simulink model "Subsystem_repository0x5B10x5D"  (R2023b)
settings: Solver=VariableStepAuto  StartTime=0.0  StopTime=10.0  RelTol=1e-3
values from neighbouring files (symbols this model uses):
  A0 = [1 0 0; 0 0 1; 0 -1 0]*[0 0 1; 0 1 0; -1 0 0]    [planetary_phase_script.m]    (also in script_aocs.m = [0 0 1; 0 1 0; -1 0 0]; script_jupiter.m; simulation_inner1.m = A_b_n(:,:,end); srp_interplanetary.m = A_b_n(:,:,end))
  mu = astroConstants(4)    [calcolo_distanze.m]    (also in loadData.m; loadData_ore.m; planetary_phase_script.m = astroConstants(15); script_aocs.m)
  toll = deg2rad(15)    [planetary_phase_script.m]    (also in script_aocs.m; script_jupiter.m; simulation_inner1.m; srp_interplanetary.m)
undefined symbols (not defined in the file or in its folder): N, q0
libraries: simulink x3, matrix_library x3, vrlib x1
(part 1 of 2)
settings Model: Creator=ricky  LastModifiedBy=paolo

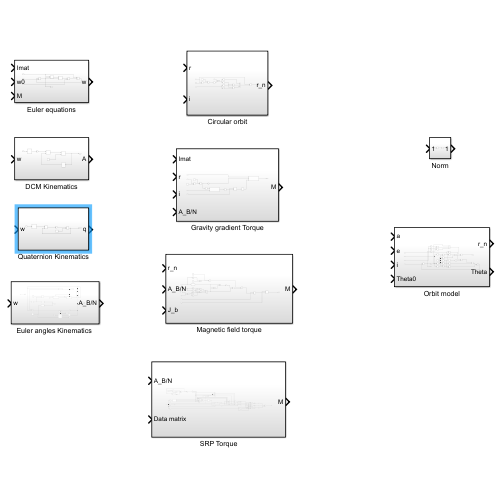
[thumbnail: Simulink's stored preview of the top-level diagram]
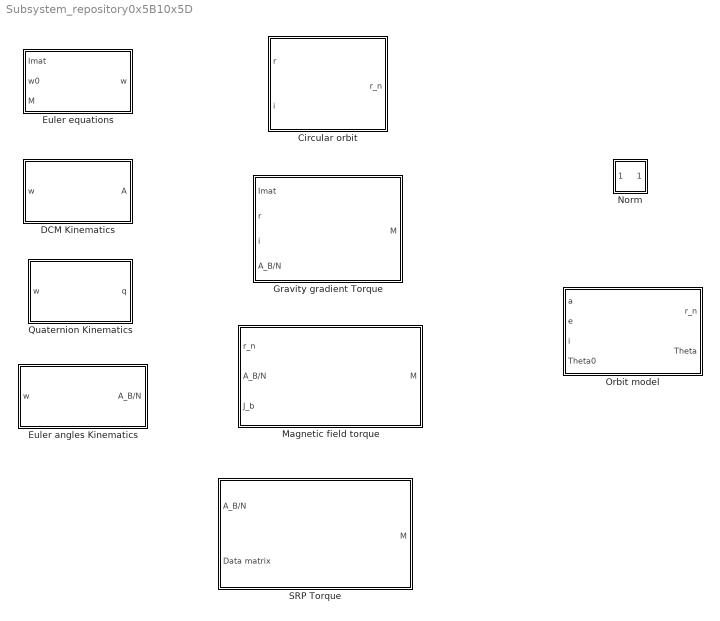
== system Subsystem_repository0x5B10x5D ==
  Circular orbit : Subsystem
  DCM Kinematics : Subsystem
  "Euler angles Kinematics " : Subsystem
  Euler equations : Subsystem
  Gravity gradient Torque : Subsystem
  Magnetic field torque : Subsystem
  Norm : Subsystem
  Orbit model : Subsystem
  Quaternion Kinematics : Subsystem
  SRP Torque : Subsystem

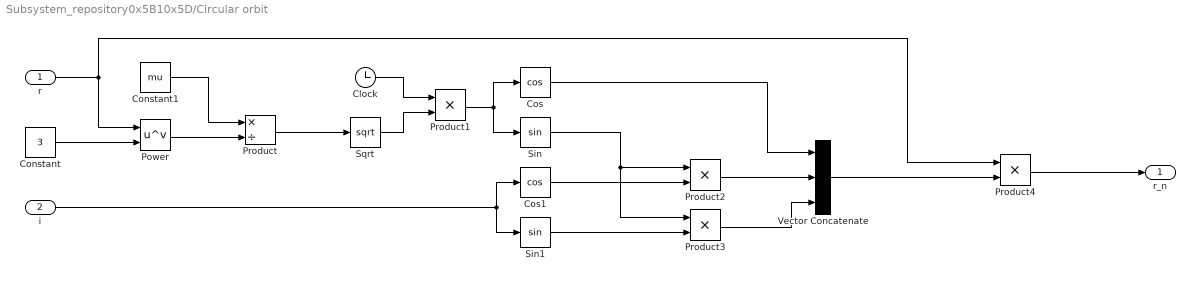
== system Subsystem_repository0x5B10x5D/Circular orbit ==
  r : Inport
  i : Inport  Port=2
  Clock : Clock
  Constant : Constant  Value=3
  Constant1 : Constant  Value=mu
  Cos : Trigonometry  Operator=cos
  Cos1 : Trigonometry  Operator=cos
  Power : Math  Operator=pow
  Product : Product  Inputs=*/
  Product{1..4} (4 alike) : Product
  Sin : Trigonometry
  Sin1 : Trigonometry
  Sqrt : Sqrt
  Vector Concatenate : Concatenate  NumInputs=3
  r_n : Outport
  wires:
  Product/1 -> Sqrt/1
  Constant/1 -> Power/2
  Constant1/1 -> Product/1
  Power/1 -> Product/2
  r/1 -> Product4/1, Power/1
  Clock/1 -> Product1/1
  Sqrt/1 -> Product1/2
  Product1/1 -> Cos/1, Sin/1
  i/1 -> Sin1/1, Cos1/1
  Product2/1 -> Vector Concatenate/2
  Product3/1 -> Vector Concatenate/3
  Cos/1 -> Vector Concatenate/1
  Sin/1 -> Product3/1, Product2/1
  Cos1/1 -> Product2/2
  Sin1/1 -> Product3/2
  Vector Concatenate/1 -> Product4/2
  Product4/1 -> r_n/1

== system Subsystem_repository0x5B10x5D/DCM Kinematics ==
  w : Inport
  Constant : Constant  Value=A0
  Gain : Gain  Gain=-1
  Integrator : Integrator  InitialConditionSource=external
  Matrix Creation : Subsystem
  Matrix orthonormalization : Subsystem
  MatrixMultiply : Product  Multiplication=Matrix(*)
  A : Outport
  wires:
  Matrix orthonormalization/1(Out1) -> MatrixMultiply/2
  Integrator/1 -> A/1, Matrix orthonormalization/1(A)  "A"
  Constant/1 -> Integrator/2
  MatrixMultiply/1 -> Integrator/1  "A_d"
  Matrix Creation/1(Out1) -> Gain/1
  Gain/1 -> MatrixMultiply/1
  w/1 -> Matrix Creation/1(Input)

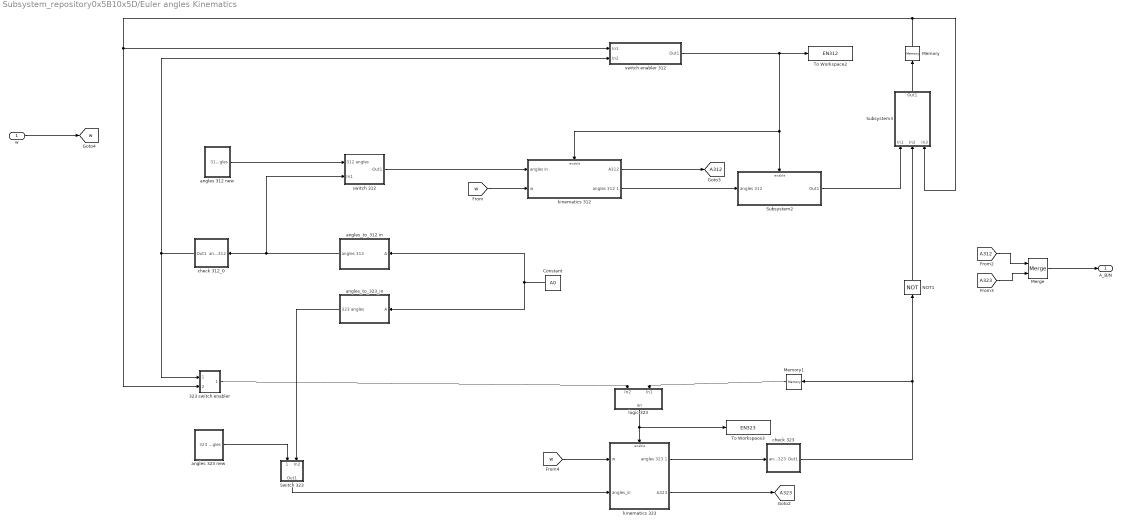
== system Subsystem_repository0x5B10x5D/Euler angles Kinematics  ==
  w : Inport
  323 switch enabler : Subsystem
  Constant : Constant  Value=A0
  Memory : Memory  InheritSampleTime=on
  Memory1 : Memory
  Merge : Merge
  NOT1 : Logic  Operator=NOT  IconShape=distinctive  AllPortsSameDT=off  OutDataTypeStr=boolean
  Subsystem2 : Subsystem
  Subsystem3 : Subsystem
  Switch 323 : Subsystem
  To Workspace2 : ToWorkspace  VariableName=EN312  SampleTime=-1
  To Workspace3 : ToWorkspace  VariableName=EN323  SampleTime=-1
  angles 312 new : Subsystem
  angles 323 new : Subsystem
  angles_to_312 in : Subsystem
  angles_to_323_in : Subsystem
  check 312_0 : Subsystem
      settings: PortSchema="{\"entries\":[{\"content\":{\"sides\":[{\"content\":{},\"type\":\"ConnectorPlacement.EquallySpacedRectSide\",\"uuid\":\"ce510fac-c30a-4239-a3ca-34d3b3a25917\"},{\"content\":{\"side\":\"RIGHT\"},\"type\":\"ConnectorPlacement.EquallySpacedRectSide\",\"uuid\":\"eef8e0af-d591-4c9d-a699-4633d685d136\"},{\"content\":{\"connectorIds\":[\"Out1\"],\"side\":\"TOP\"},\"type\":\"ConnectorPlacement.EquallySpacedRectSide\",\"uuid\":\"fcaa08d0-a3a1-4dce-b64a-8b5dfd06733d\"},{\"content\":{\"connectorIds\":[\"In1\"],\"side\":\"BOTTOM\"},\"type\":\"ConnectorPlacement.EquallySpacedRectSide\",\"uuid\":\"e9ea2ab9-2ba0-4219-9d61-f42bbc501f13\"}]},\"type\":\"ConnectorPlacement.EquallySpacedConnector\",\"uuid\":\"4537d4ba-38a8-4a93-90f3-8d5d5085984b\"}],\"packageUris\":[\"http://schema.mathworks.com/mf0/Connector/R2020b\"],\"version\":\"1.0\"}"
  check 323 : Subsystem
      settings: PortSchema="{\"entries\":[{\"content\":{\"sides\":[{\"content\":{},\"type\":\"ConnectorPlacement.EquallySpacedRectSide\",\"uuid\":\"ce510fac-c30a-4239-a3ca-34d3b3a25917\"},{\"content\":{\"side\":\"RIGHT\"},\"type\":\"ConnectorPlacement.EquallySpacedRectSide\",\"uuid\":\"eef8e0af-d591-4c9d-a699-4633d685d136\"},{\"content\":{\"connectorIds\":[\"Out1\"],\"side\":\"TOP\"},\"type\":\"ConnectorPlacement.EquallySpacedRectSide\",\"uuid\":\"fcaa08d0-a3a1-4dce-b64a-8b5dfd06733d\"},{\"content\":{\"connectorIds\":[\"In1\"],\"side\":\"BOTTOM\"},\"type\":\"ConnectorPlacement.EquallySpacedRectSide\",\"uuid\":\"e9ea2ab9-2ba0-4219-9d61-f42bbc501f13\"}]},\"type\":\"ConnectorPlacement.EquallySpacedConnector\",\"uuid\":\"4537d4ba-38a8-4a93-90f3-8d5d5085984b\"}],\"packageUris\":[\"http://schema.mathworks.com/mf0/Connector/R2020b\"],\"version\":\"1.0\"}"
  kinematics 312 : Subsystem
  kinematics 323 : Subsystem
  logic 323 : Subsystem
  switch 312 : Subsystem
  switch enabler 312 : Subsystem
  A_B/N : Outport
  tag scope: A312=global, A323=global, w=global
  wires:
  kinematics 323/2(A323) -> [A323]
  Constant/1 -> angles_to_323_in/1(A), angles_to_312 in/1(A)
  323 switch enabler/1(Out1) -> logic 323/1(In2)
  logic 323/1(en) -> To Workspace3/1, kinematics 323/Enable
  switch enabler 312/1(Out1) -> To Workspace2/1, Subsystem2/Enable, kinematics 312/Enable
  kinematics 312/2(angles 312 1) -> Subsystem2/1(angles 312)
  check 312_0/1(Out1) -> switch enabler 312/2(In2), 323 switch enabler/1(In2)
  [w] -> kinematics 323/1(w)
  angles_to_312 in/1(angles 312) -> switch 312/2(In1), check 312_0/1(angles 312)
  Memory1/1 -> logic 323/2(In1)
  Subsystem3/1(Out1) -> Memory/1
  w/1 -> [w]
  NOT1/1 -> Subsystem3/2(In2)
  Memory/1 -> Subsystem3/3(In3), 323 switch enabler/2(In1), switch enabler 312/1(In1)
  kinematics 323/1(angles 323 1) -> check 323/1(angles 323)
  kinematics 312/1(A312) -> [A312]
  switch 312/1(Out1) -> kinematics 312/1(angles in)
  Merge/1 -> A_B/N/1
  Switch 323/1(Out1) -> kinematics 323/2(angles_in)
  check 323/1(Out1) -> NOT1/1, Memory1/1
  Subsystem2/1(Out1) -> Subsystem3/1(In1)
  angles 323 new/1(323 angles) -> Switch 323/1(323 angles)
  angles 312 new/1(312 angles) -> switch 312/1(312 angles)
  [w] -> kinematics 312/2(w)
  angles_to_323_in/1(323 angles) -> Switch 323/2(In2)
  [A323] -> Merge/2
  [A312] -> Merge/1

== system Subsystem_repository0x5B10x5D/Euler equations ==
  Imat : Inport
  w0 : Inport  Port=2
  M : Inport  Port=3
  Cross Product : matrix_library/Cross Product
  Integrator1 : Integrator  InitialConditionSource=external
  Product : Product  Multiplication=Matrix(*)
  Product1 : Product  Inputs=/*  Multiplication=Matrix(*)
  Subtract : Sum
  w : Outport
  wires:
  Imat/1 -> Product1/1, Product/1
  Integrator1/1 -> w/1, Product/2, Cross Product/2  "w"
  Product/1 -> Cross Product/1
  w0/1 -> Integrator1/2
  Cross Product/1 -> Subtract/1
  M/1 -> Subtract/2
  Subtract/1 -> Product1/2
  Product1/1 -> Integrator1/1

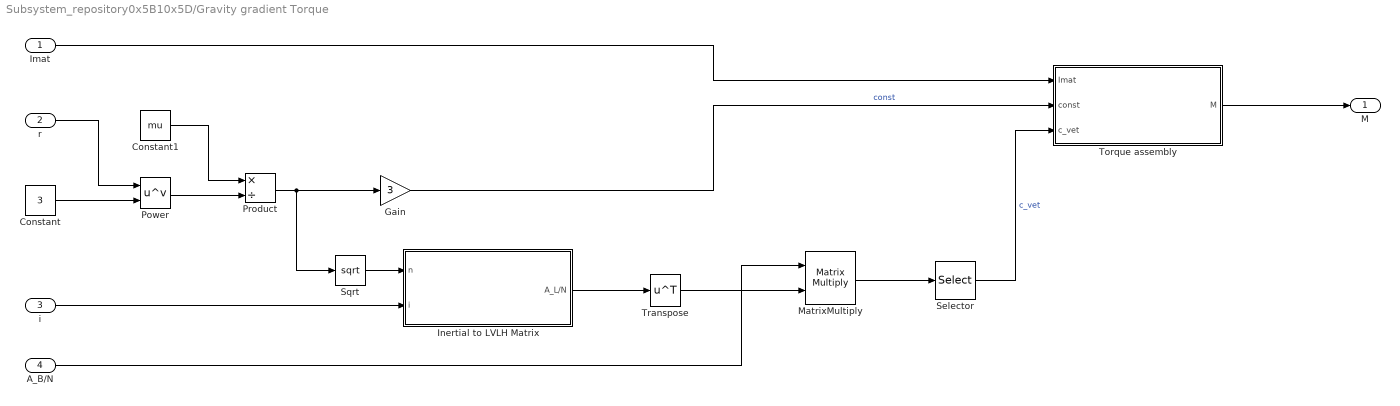
== system Subsystem_repository0x5B10x5D/Gravity gradient Torque ==
  Imat : Inport
  r : Inport  Port=2
  i : Inport  Port=3
  A_B/N : Inport  Port=4
  Constant : Constant  Value=3
  Constant1 : Constant  Value=mu
  Gain : Gain  Gain=3
  Inertial to LVLH Matrix : Subsystem
  MatrixMultiply : Product  Multiplication=Matrix(*)
  Power : Math  Operator=pow
  Product : Product  Inputs=*/
  Selector : Selector  NumberOfDimensions=2  InputPortWidth=3  IndexOptions=Index vector (dialog),Index vector (dialog)  Indices=[1 2 3],1  OutputSizes=1,1
  Sqrt : Sqrt
  Torque assembly : Subsystem
  Transpose : Math  Operator=transpose
  M : Outport
  wires:
  Inertial to LVLH Matrix/1(A_L/N) -> Transpose/1
  Transpose/1 -> MatrixMultiply/2
  MatrixMultiply/1 -> Selector/1
  i/1 -> Inertial to LVLH Matrix/2(i)
  A_B/N/1 -> MatrixMultiply/1
  Power/1 -> Product/2
  r/1 -> Power/1
  Constant/1 -> Power/2
  Product/1 -> Sqrt/1, Gain/1
  Constant1/1 -> Product/1
  Sqrt/1 -> Inertial to LVLH Matrix/1(n)
  Selector/1 -> Torque assembly/3(c_vet)  "c_vet"
  Gain/1 -> Torque assembly/2(const)  "const"
  Imat/1 -> Torque assembly/1(Imat)
  Torque assembly/1(M) -> M/1

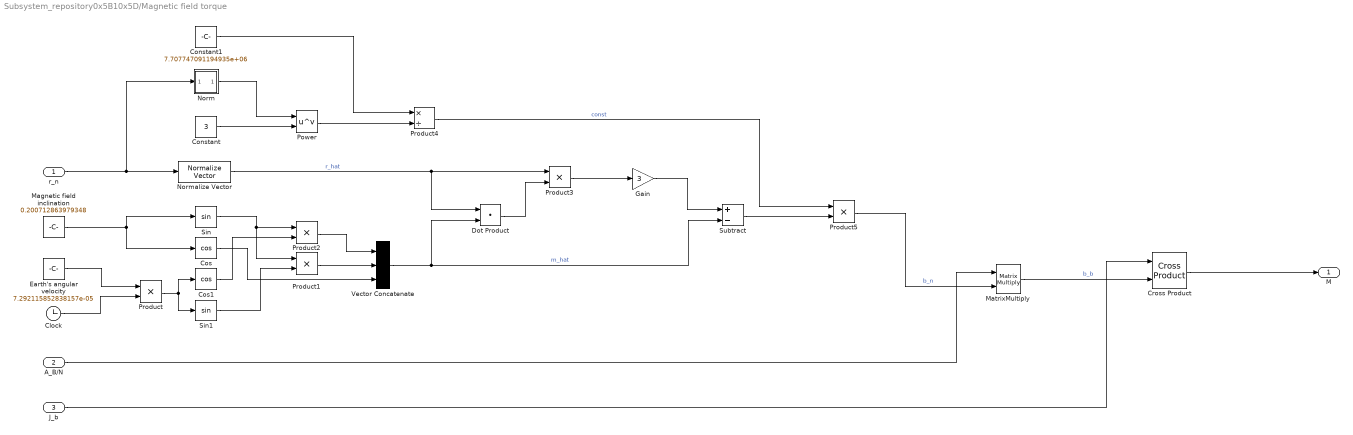
== system Subsystem_repository0x5B10x5D/Magnetic field torque ==
  r_n : Inport
  A_B/N : Inport  Port=2
  J_b : Inport  Port=3
  Clock : Clock
  Constant : Constant  Value=3
  Constant1 : Constant  Value=7.707747091194935e+06
  Cos : Trigonometry  Operator=cos
  Cos1 : Trigonometry  Operator=cos
  Cross Product : matrix_library/Cross Product
  Dot Product : DotProduct  OutDataTypeStr=Inherit: Inherit via internal rule
  Earth's angular velocity : Constant  Value=7.292115852838157e-05
  Gain : Gain  Gain=3
  Magnetic field inclination : Constant  Value=0.200712863979348
  MatrixMultiply : Product  Multiplication=Matrix(*)
  Norm : Subsystem
  Normalize Vector : vrlib/Utilities/Normalize Vector  maxzero=0
  Power : Math  Operator=pow
  Product{,1..3,5} (5 alike) : Product
  Product4 : Product  Inputs=*/
  Sin : Trigonometry
  Sin1 : Trigonometry
  Subtract : Sum  Inputs=+-
  Vector Concatenate : Concatenate  NumInputs=3
  M : Outport
  wires:
  r_n/1 -> Norm/1(1), Normalize Vector/1
  Normalize Vector/1 -> Product3/1, Dot Product/1  "r_hat"
  Earth's angular velocity/1 -> Product/1
  Clock/1 -> Product/2
  Product/1 -> Sin1/1, Cos1/1
  Magnetic field inclination/1 -> Cos/1, Sin/1
  Cos/1 -> Vector Concatenate/3
  Product1/1 -> Vector Concatenate/2
  Product2/1 -> Vector Concatenate/1
  Sin/1 -> Product1/1, Product2/1
  Cos1/1 -> Product2/2
  Sin1/1 -> Product1/2
  Vector Concatenate/1 -> Subtract/2, Dot Product/2  "m_hat"
  Dot Product/1 -> Product3/2
  Product3/1 -> Gain/1
  Gain/1 -> Subtract/1
  A_B/N/1 -> MatrixMultiply/1
  MatrixMultiply/1 -> Cross Product/2  "b_b"
  J_b/1 -> Cross Product/1
  Constant1/1 -> Product4/1
  Subtract/1 -> Product5/2
  Product4/1 -> Product5/1  "const"
  Product5/1 -> MatrixMultiply/2  "b_n"
  Cross Product/1 -> M/1
  Constant/1 -> Power/2
  Power/1 -> Product4/2
  Norm/1(Output) -> Power/1

== system Subsystem_repository0x5B10x5D/Norm ==
  1 : Inport
  Dot Product : DotProduct  OutDataTypeStr=Inherit: Inherit via internal rule
  Sqrt : Sqrt
  Output : Outport
  wires:
  1/1 -> Dot Product/1, Dot Product/2
  Dot Product/1 -> Sqrt/1
  Sqrt/1 -> Output/1

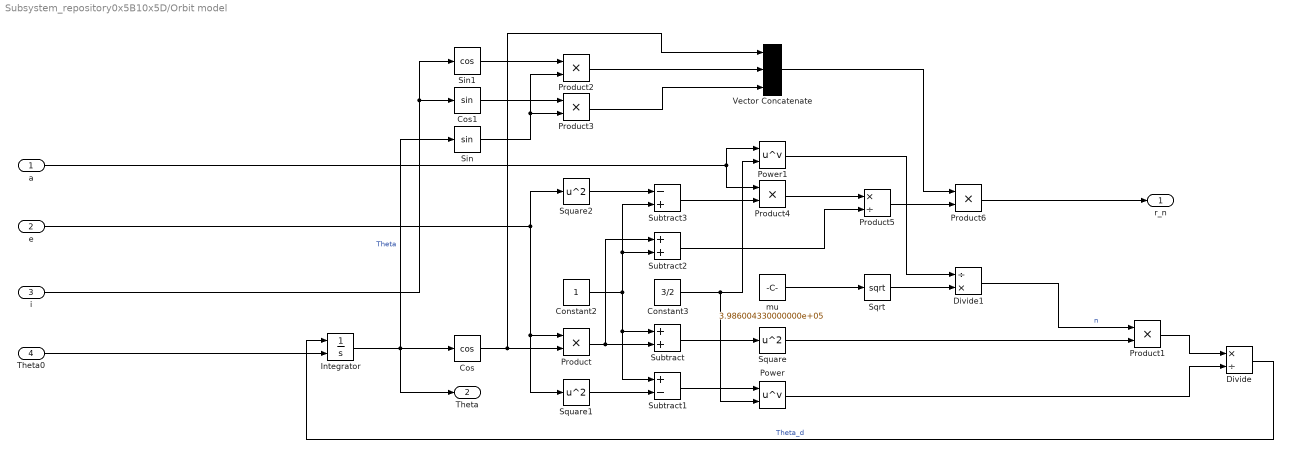
== system Subsystem_repository0x5B10x5D/Orbit model ==
  a : Inport
  e : Inport  Port=2
  i : Inport  Port=3
  Theta0 : Inport  Port=4
  Constant2 : Constant
  Constant3 : Constant  Value=3/2
  Cos : Trigonometry  Operator=cos
  Cos1 : Trigonometry
  Divide : Product  Inputs=*/
  Divide1 : Product  Inputs=/*
  Integrator : Integrator  InitialConditionSource=external
  Power : Math  Operator=pow
  Power1 : Math  Operator=pow
  Product{,1..4,6} (6 alike) : Product
  Product5 : Product  Inputs=*/
  Sin : Trigonometry
  Sin1 : Trigonometry  Operator=cos
  Sqrt : Sqrt
  Square : Math  Operator=square
  Square1 : Math  Operator=square
  Square2 : Math  Operator=square
  Subtract : Sum
  Subtract1 : Sum  Inputs=+-
  Subtract2 : Sum
  Subtract3 : Sum  Inputs=-+
  Vector Concatenate : Concatenate  NumInputs=3
  mu : Constant  Value=3.986004330000000e+05
  r_n : Outport
  Theta : Outport  Port=2
  wires:
  Constant3/1 -> Power1/2, Power/2
  Product5/1 -> Product6/2
  Power1/1 -> Divide1/1
  Subtract3/1 -> Product4/2
  Subtract2/1 -> Product5/2
  Theta0/1 -> Integrator/2
  Cos/1 -> Vector Concatenate/1, Product/2
  Subtract/1 -> Square/1
  Product/1 -> Subtract2/1, Subtract/2
  a/1 -> Power1/1, Product4/1
  Sin/1 -> Product3/2, Product2/2
  Divide/1 -> Integrator/1  "Theta_d"
  Sin1/1 -> Product2/1
  Square1/1 -> Subtract1/2
  e/1 -> Square2/1, Square1/1, Product/1
  Product4/1 -> Product5/1
  Product1/1 -> Divide/1
  Subtract1/1 -> Power/1
  Vector Concatenate/1 -> Product6/1
  Product3/1 -> Vector Concatenate/3
  Sqrt/1 -> Divide1/2
  Integrator/1 -> Theta/1, Sin/1, Cos/1  "Theta"
  Square/1 -> Product1/2
  Product2/1 -> Vector Concatenate/2
  i/1 -> Sin1/1, Cos1/1
  Square2/1 -> Subtract3/1
  Cos1/1 -> Product3/1
  Power/1 -> Divide/2
  Constant2/1 -> Subtract3/2, Subtract2/2, Subtract1/1, Subtract/1
  Divide1/1 -> Product1/1  "n"
  Product6/1 -> r_n/1
  mu/1 -> Sqrt/1

== system Subsystem_repository0x5B10x5D/Quaternion Kinematics ==
  w : Inport
  Constant : Constant  Value=q0
  Gain : Gain  Gain=1/2
  Integrator : Integrator  InitialConditionSource=external
  Matrix creation : Subsystem
  Product : Product  Multiplication=Matrix(*)
  q : Outport
  wires:
  Matrix creation/1(Out1) -> Product/1  "wmat"
  Integrator/1 -> q/1, Product/2  "q"
  Gain/1 -> Integrator/1
  Product/1 -> Gain/1  "q_d"
  Constant/1 -> Integrator/2
  w/1 -> Matrix creation/1(In1)

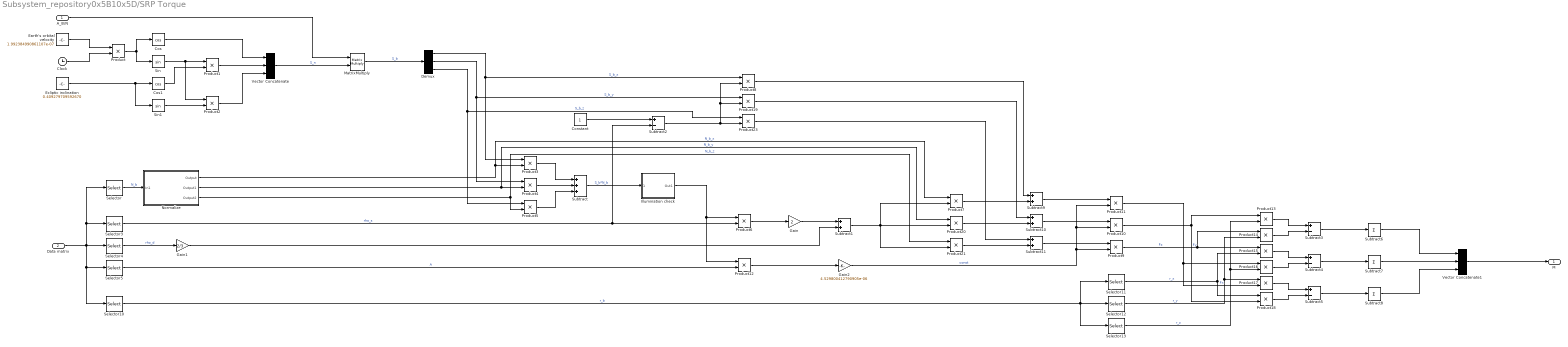
== system Subsystem_repository0x5B10x5D/SRP Torque ==
  A_B/N : Inport
  Data matrix : Inport  Port=2
  Clock : Clock
  Constant : Constant
  Cos : Trigonometry  Operator=cos
  Cos1 : Trigonometry  Operator=cos
  Demux : Demux  Outputs=3
  Earth's orbital velocity : Constant  Value=1.992384990861107e-07
  Ecliptic inclination : Constant  Value=0.409279709592670
  Gain : Gain  Gain=2
  Gain1 : Gain  Gain=2/3
  Gain2 : Gain  Gain=4.529800412790905e-06
  Illumination check : Subsystem
  MatrixMultiply : Product  Multiplication=Matrix(*)
  Normalize : Subsystem
  Product{,1..21,23} (23 alike) : Product
  Selector : Selector  NumberOfDimensions=2  InputPortWidth=3  IndexOptions=Index vector (dialog),Index vector (dialog)  Indices=1:N,1:3  OutputSizes=1,1
  Selector10 : Selector  NumberOfDimensions=2  InputPortWidth=3  IndexOptions=Index vector (dialog),Index vector (dialog)  Indices=1:N,7:9  OutputSizes=1,1
  Selector11 : Selector  NumberOfDimensions=2  InputPortWidth=3  IndexOptions=Index vector (dialog),Index vector (dialog)  Indices=1:N,1  OutputSizes=1,1
  Selector12 : Selector  NumberOfDimensions=2  InputPortWidth=3  IndexOptions=Index vector (dialog),Index vector (dialog)  Indices=1:N,2  OutputSizes=1,1
  Selector13 : Selector  NumberOfDimensions=2  InputPortWidth=3  IndexOptions=Index vector (dialog),Index vector (dialog)  Indices=1:N,3  OutputSizes=1,1
  Selector3 : Selector  NumberOfDimensions=2  InputPortWidth=3  IndexOptions=Index vector (dialog),Index vector (dialog)  Indices=1:N,4  OutputSizes=1,1
  Selector4 : Selector  NumberOfDimensions=2  InputPortWidth=3  IndexOptions=Index vector (dialog),Index vector (dialog)  Indices=1:N,5  OutputSizes=1,1
  Selector5 : Selector  NumberOfDimensions=2  InputPortWidth=3  IndexOptions=Index vector (dialog),Index vector (dialog)  Indices=1:N,6  OutputSizes=1,1
  Sin : Trigonometry
  Sin1 : Trigonometry
  Subtract : Sum  Inputs=+++
  Subtract{1,9..11} (4 alike) : Sum
  Subtract{2..5} (4 alike) : Sum  Inputs=+-
  Subtract6 : Sum  Inputs=+
  Subtract7 : Sum  Inputs=+
  Subtract8 : Sum  Inputs=+
  Vector Concatenate : Concatenate  NumInputs=3
  Vector Concatenate1 : Concatenate  NumInputs=3
  M : Outport
  wires:
  Earth's orbital velocity/1 -> Product/1
  Clock/1 -> Product/2
  Product/1 -> Sin/1, Cos/1
  Ecliptic inclination/1 -> Sin1/1, Cos1/1
  Sin/1 -> Product2/1, Product1/1
  Cos1/1 -> Product1/2
  Sin1/1 -> Product2/2
  Product1/1 -> Vector Concatenate/2
  Product2/1 -> Vector Concatenate/3
  Cos/1 -> Vector Concatenate/1
  Vector Concatenate/1 -> MatrixMultiply/2  "S_n"
  A_B/N/1 -> MatrixMultiply/1
  MatrixMultiply/1 -> Demux/1  "S_b"
  Data matrix/1 -> Selector/1, Selector3/1, Selector10/1, Selector5/1, Selector4/1
  Demux/1 -> Product3/1, Product8/1  "S_b_x"
  Demux/2 -> Product4/1, Product19/1  "S_b_y"
  Demux/3 -> Product23/1, Product5/1  "S_b_z"
  Product4/1 -> Subtract/2
  Product3/1 -> Subtract/1
  Product5/1 -> Subtract/3
  Subtract/1 -> Illumination check/1(1)  "S_b*N_b"
  Illumination check/1(Out1) -> Product12/1, Product6/1
  Selector4/1 -> Gain1/1  "rho_d"
  Selector5/1 -> Product12/2  "A"
  Normalize/1(Output) -> Product7/1, Product3/2  "N_b_x"
  Normalize/2(Output1) -> Product20/1, Product4/2  "N_b_y"
  Normalize/3(Output2) -> Product21/1, Product5/2  "N_b_z"
  Product6/1 -> Gain/1
  Selector3/1 -> Product6/2, Subtract2/2  "rho_s"
  Gain1/1 -> Subtract1/2
  Gain/1 -> Subtract1/1
  Constant/1 -> Subtract2/1
  Subtract2/1 -> Product8/2, Product19/2, Product23/2
  Product12/1 -> Gain2/1
  Selector10/1 -> Selector13/1, Selector11/1, Selector12/1  "r_b"
  Product13/1 -> Subtract3/1
  Product14/1 -> Subtract3/2
  Product16/1 -> Subtract4/2
  Product15/1 -> Subtract4/1
  Product18/1 -> Subtract5/2
  Product17/1 -> Subtract5/1
  Subtract5/1 -> Subtract8/1
  Subtract4/1 -> Subtract7/1
  Subtract3/1 -> Subtract6/1
  Subtract7/1 -> Vector Concatenate1/2
  Subtract6/1 -> Vector Concatenate1/1
  Subtract8/1 -> Vector Concatenate1/3
  Vector Concatenate1/1 -> M/1
  Subtract1/1 -> Product20/2, Product7/2, Product21/2
  Product7/1 -> Subtract9/2
  Product21/1 -> Subtract11/2
  Product20/1 -> Subtract10/2
  Subtract9/1 -> Product11/1
  Subtract10/1 -> Product10/1
  Subtract11/1 -> Product9/1
  Gain2/1 -> Product10/2, Product11/2, Product9/2  "const"
  Product8/1 -> Subtract9/1
  Product19/1 -> Subtract10/1
  Product23/1 -> Subtract11/1
  Product11/1 -> Product17/2, Product16/1  "Fx"
  Product10/1 -> Product18/2, Product13/1  "Fy"
  Product9/1 -> Product14/1, Product15/1  "Fz"
  Selector11/1 -> Product15/2, Product18/1  "r_x"
  Selector12/1 -> Product17/1, Product14/2  "r_y"
  Selector13/1 -> Product16/2, Product13/2  "r_z"
  Selector/1 -> Normalize/1(In1)  "N_b"

== system Subsystem_repository0x5B10x5D/DCM Kinematics/Matrix Creation ==
  Input : Inport
  Constant : Constant  Value=0
  Demux : Demux  Outputs=3
      settings: DisplayOption=none
  Gain : Gain  Gain=-1
  Gain1 : Gain  Gain=-1
  Gain2 : Gain  Gain=-1
  Reshape : Reshape
  Vector Concatenate : Concatenate  NumInputs=3
  Vector Concatenate1 : Concatenate  NumInputs=3
  Vector Concatenate2 : Concatenate  NumInputs=3
  Vector Concatenate3 : Concatenate  NumInputs=3  Mode=Multidimensional array  ConcatenateDimension=2
  Out1 : Outport
  wires:
  Constant/1 -> Vector Concatenate/1, Vector Concatenate1/2, Vector Concatenate2/3
  Demux/1 -> Gain2/1, Vector Concatenate1/3
  Vector Concatenate/1 -> Vector Concatenate3/1
  Gain/1 -> Vector Concatenate/3
  Vector Concatenate2/1 -> Vector Concatenate3/3
  Vector Concatenate1/1 -> Vector Concatenate3/2
  Demux/3 -> Gain1/1, Vector Concatenate/2
  Gain1/1 -> Vector Concatenate1/1
  Demux/2 -> Gain/1, Vector Concatenate2/1
  Gain2/1 -> Vector Concatenate2/2
  Vector Concatenate3/1 -> Out1/1
  Input/1 -> Demux/1

== system Subsystem_repository0x5B10x5D/DCM Kinematics/Matrix orthonormalization ==
  A : Inport
  Gain : Gain  Gain=1.5
  Gain1 : Gain  Gain=0.5
  MatrixMultiply1 : Product  Inputs=3  Multiplication=Matrix(*)
  Subtract : Sum  Inputs=+-
  Transpose : Math  Operator=transpose
  Out1 : Outport
  wires:
  A/1 -> Gain/1, MatrixMultiply1/1, Transpose/1, Gain1/1
  Transpose/1 -> MatrixMultiply1/2
  Gain1/1 -> MatrixMultiply1/3
  Gain/1 -> Subtract/1
  MatrixMultiply1/1 -> Subtract/2
  Subtract/1 -> Out1/1

== system Subsystem_repository0x5B10x5D/Euler angles Kinematics /323 switch enabler ==
  In2 : Inport
  In1 : Inport  Port=2
  Clock2 : Clock
  NOT : Logic  Operator=NOT  IconShape=distinctive  AllPortsSameDT=off  OutDataTypeStr=boolean
  Switch2 : Switch  Criteria=u2 > Threshold  SaturateOnIntegerOverflow=off  InputSameDT=off
  Out1 : Outport
  wires:
  Switch2/1 -> NOT/1
  In2/1 -> Switch2/3
  Clock2/1 -> Switch2/2
  In1/1 -> Switch2/1
  NOT/1 -> Out1/1

== system Subsystem_repository0x5B10x5D/Euler angles Kinematics /Subsystem2 ==
  angles 312 : Inport
  Enable : EnablePort
  check 312_1 : Subsystem
      settings: PortSchema="{\"entries\":[{\"content\":{\"sides\":[{\"content\":{},\"type\":\"ConnectorPlacement.EquallySpacedRectSide\",\"uuid\":\"ce510fac-c30a-4239-a3ca-34d3b3a25917\"},{\"content\":{\"side\":\"RIGHT\"},\"type\":\"ConnectorPlacement.EquallySpacedRectSide\",\"uuid\":\"eef8e0af-d591-4c9d-a699-4633d685d136\"},{\"content\":{\"connectorIds\":[\"Out1\"],\"side\":\"TOP\"},\"type\":\"ConnectorPlacement.EquallySpacedRectSide\",\"uuid\":\"fcaa08d0-a3a1-4dce-b64a-8b5dfd06733d\"},{\"content\":{\"connectorIds\":[\"In1\"],\"side\":\"BOTTOM\"},\"type\":\"ConnectorPlacement.EquallySpacedRectSide\",\"uuid\":\"e9ea2ab9-2ba0-4219-9d61-f42bbc501f13\"}]},\"type\":\"ConnectorPlacement.EquallySpacedConnector\",\"uuid\":\"4537d4ba-38a8-4a93-90f3-8d5d5085984b\"}],\"packageUris\":[\"http://schema.mathworks.com/mf0/Connector/R2020b\"],\"version\":\"1.0\"}"
  Out1 : Outport
  wires:
  angles 312/1 -> check 312_1/1(angles 312)
  check 312_1/1(Out1) -> Out1/1

== system Subsystem_repository0x5B10x5D/Euler angles Kinematics /Subsystem3 ==
  In1 : Inport
  In2 : Inport  Port=2
  In3 : Inport  Port=3
  Constant : Constant
  Constant1 : Constant
  Constant2 : Constant  Value=0
  Constant3 : Constant  Value=0
  Data Type Conversion : DataTypeConversion  OutDataTypeStr=boolean  SaturateOnIntegerOverflow=off  RndMeth=Floor
  If Action Subsystem : Subsystem  TreatAsAtomicUnit=on
  If Action Subsystem1 : Subsystem  TreatAsAtomicUnit=on
  If Action Subsystem2 : Subsystem  TreatAsAtomicUnit=on
  If Action Subsystem3 : Subsystem  TreatAsAtomicUnit=on
  If2 : If  NumInputs=3  IfExpression=u1 == 1  ElseIfExpressions=u1 == 0 & u2 == 1 & u3 == 1, u1 == 0 & u2 == 1 & u3 == 0
  Merge : Merge  Inputs=4
  Out1 : Outport
  wires:
  In2/1 -> If2/2
  In1/1 -> If2/1
  In3/1 -> If2/3
  If2/1 -> If Action Subsystem/Action
  If2/2 -> If Action Subsystem1/Action
  If2/3 -> If Action Subsystem2/Action
  If2/4 -> If Action Subsystem3/Action
  Constant/1 -> If Action Subsystem/1(In1)
  Constant1/1 -> If Action Subsystem2/1(In1)
  Constant2/1 -> If Action Subsystem1/1(In1)
  Constant3/1 -> If Action Subsystem3/1(In1)
  If Action Subsystem/1(Out1) -> Merge/1
  If Action Subsystem1/1(Out1) -> Merge/2
  If Action Subsystem2/1(Out1) -> Merge/3
  If Action Subsystem3/1(Out1) -> Merge/4
  Merge/1 -> Data Type Conversion/1
  Data Type Conversion/1 -> Out1/1

== system Subsystem_repository0x5B10x5D/Euler angles Kinematics /Switch 323 ==
  323 angles : Inport
  In2 : Inport  Port=2
  Clock3 : Clock
  Switch3 : Switch  Criteria=u2 > Threshold  SaturateOnIntegerOverflow=off  InputSameDT=off
  Out1 : Outport
  wires:
  Clock3/1 -> Switch3/2
  In2/1 -> Switch3/3
  323 angles/1 -> Switch3/1
  Switch3/1 -> Out1/1

== system Subsystem_repository0x5B10x5D/Euler angles Kinematics /angles 312 new ==
  A323 matrix : Subsystem
  angles_to_312 : Subsystem
  312 angles : Outport
  wires:
  [phi323] -> A323 matrix/1(phi)
  [theta323] -> A323 matrix/2(theta)
  [psi323] -> A323 matrix/3(psi)
  angles_to_312/1(312 angles) -> 312 angles/1
  A323 matrix/1(A323) -> angles_to_312/1(A323)

== system Subsystem_repository0x5B10x5D/Euler angles Kinematics /angles 323 new ==
  Rotation 312 matrix2 : Subsystem
  angles_to_323 : Subsystem
  323 angles : Outport
  wires:
  [theta312] -> Rotation 312 matrix2/2(theta)
  [psi_312] -> Rotation 312 matrix2/3(psi)
  Rotation 312 matrix2/1(A312) -> angles_to_323/1(A312)
  [phi312] -> Rotation 312 matrix2/1(phi)
  angles_to_323/1(323 angles) -> 323 angles/1

== system Subsystem_repository0x5B10x5D/Euler angles Kinematics /angles_to_312 in ==
  A : Inport
  Asin : Trigonometry  Operator=asin
  Atan1 : Trigonometry  Operator=atan2
  Atan2 : Trigonometry  Operator=atan2
  Gain : Gain  Gain=-1
  Gain1 : Gain  Gain=-1
  Mux : Mux  Inputs=3
  Selector : Selector  NumberOfDimensions=2  InputPortWidth=3  IndexOptions=Index vector (dialog),Index vector (dialog)  Indices=2,1  OutputSizes=1,1
  Selector1 : Selector  NumberOfDimensions=2  InputPortWidth=3  IndexOptions=Index vector (dialog),Index vector (dialog)  Indices=2,2  OutputSizes=1,1
  Selector2 : Selector  NumberOfDimensions=2  InputPortWidth=3  IndexOptions=Index vector (dialog),Index vector (dialog)  Indices=2,3  OutputSizes=1,1
  Selector3 : Selector  NumberOfDimensions=2  InputPortWidth=3  IndexOptions=Index vector (dialog),Index vector (dialog)  Indices=1,3  OutputSizes=1,1
  Selector4 : Selector  NumberOfDimensions=2  InputPortWidth=3  IndexOptions=Index vector (dialog),Index vector (dialog)  Indices=3,3  OutputSizes=1,1
  angles 312 : Outport
  wires:
  Selector/1 -> Gain/1
  Gain/1 -> Atan2/1
  Selector1/1 -> Atan2/2
  Selector2/1 -> Asin/1
  Atan2/1 -> Mux/1
  Asin/1 -> Mux/2
  Mux/1 -> angles 312/1
  A/1 -> Selector3/1, Selector4/1, Selector2/1, Selector/1, Selector1/1
  Selector3/1 -> Gain1/1
  Gain1/1 -> Atan1/1
  Selector4/1 -> Atan1/2
  Atan1/1 -> Mux/3

== system Subsystem_repository0x5B10x5D/Euler angles Kinematics /angles_to_323_in ==
  A : Inport
  Asin : Trigonometry  Operator=acos
  Atan1 : Trigonometry  Operator=atan2
  Atan2 : Trigonometry  Operator=atan2
  Gain2 : Gain  Gain=-1
  Mux : Mux  Inputs=3
  Selector : Selector  NumberOfDimensions=2  InputPortWidth=3  IndexOptions=Index vector (dialog),Index vector (dialog)  Indices=3,2  OutputSizes=1,1
  Selector1 : Selector  NumberOfDimensions=2  InputPortWidth=3  IndexOptions=Index vector (dialog),Index vector (dialog)  Indices=3,1  OutputSizes=1,1
  Selector2 : Selector  NumberOfDimensions=2  InputPortWidth=3  IndexOptions=Index vector (dialog),Index vector (dialog)  Indices=3,3  OutputSizes=1,1
  Selector3 : Selector  NumberOfDimensions=2  InputPortWidth=3  IndexOptions=Index vector (dialog),Index vector (dialog)  Indices=2,3  OutputSizes=1,1
  Selector4 : Selector  NumberOfDimensions=2  InputPortWidth=3  IndexOptions=Index vector (dialog),Index vector (dialog)  Indices=1,3  OutputSizes=1,1
  323 angles : Outport
  wires:
  Gain2/1 -> Atan1/2
  Selector1/1 -> Atan2/2
  Selector2/1 -> Asin/1
  Selector/1 -> Atan2/1
  A/1 -> Selector2/1, Selector4/1, Selector3/1, Selector1/1, Selector/1
  Atan1/1 -> Mux/3
  Atan2/1 -> Mux/1
  Selector4/1 -> Gain2/1
  Selector3/1 -> Atan1/1
  Asin/1 -> Mux/2
  Mux/1 -> 323 angles/1

== system Subsystem_repository0x5B10x5D/Euler angles Kinematics /check 312_0 ==
  angles 312 : Inport
  Check Static Range : simulink/Model Verification/Check  Static Range  Description=-pi/2+toll <= u <= pi/2 - toll  max=pi/2 - toll  max_included=on  min=-pi/2+toll  min_included=on  enabled=off  stopWhenAssertionFail=off  export=on  icon=graphic
  Data Type Conversion : DataTypeConversion  OutDataTypeStr=boolean  SaturateOnIntegerOverflow=off  RndMeth=Floor
  Selector : Selector  InputPortWidth=3  IndexOptions=Index vector (dialog)  Indices=[2]  OutputSizes=1
  Out1 : Outport
  wires:
  angles 312/1 -> Selector/1
  Selector/1 -> Check Static Range/1
  Check Static Range/1 -> Data Type Conversion/1
  Data Type Conversion/1 -> Out1/1

== system Subsystem_repository0x5B10x5D/Euler angles Kinematics /check 323 ==
  angles 323 : Inport
  Check Static Range : simulink/Model Verification/Check  Static Range  Description=toll <= u <= pi - toll  max=pi - toll  max_included=on  min=toll  min_included=on  enabled=off  stopWhenAssertionFail=off  export=on  icon=graphic
  Selector : Selector  InputPortWidth=3  IndexOptions=Index vector (dialog)  Indices=2  OutputSizes=1
  Out1 : Outport
  wires:
  Check Static Range/1 -> Out1/1
  Selector/1 -> Check Static Range/1
  angles 323/1 -> Selector/1

== system Subsystem_repository0x5B10x5D/Euler angles Kinematics /kinematics 312 ==
  angles in : Inport
  w : Inport  Port=2
  Enable : EnablePort  StatesWhenEnabling=reset  ShowOutputPort=on
  Kinematics 312 : Subsystem
      settings: PortSchema="{\"entries\":[{\"content\":{\"sides\":[{\"content\":{\"connectorIds\":[\"In1\",\"In2\"]},\"type\":\"ConnectorPlacement.EquallySpacedRectSide\",\"uuid\":\"4fd6e809-7da2-4d51-96c7-4627657bb0a7\"},{\"content\":{\"connectorIds\":[\"Out1\"],\"side\":\"RIGHT\"},\"type\":\"ConnectorPlacement.EquallySpacedRectSide\",\"uuid\":\"c66e7720-5f48-4c1c-aaff-2c7b43e45843\"},{\"content\":{\"connectorIds\":[\"In3\"],\"side\":\"TOP\"},\"type\":\"ConnectorPlacement.EquallySpacedRectSide\",\"uuid\":\"5add9d35-dacd-40f3-b2c8-04b7016dc331\"}]},\"type\":\"ConnectorPlacement.EquallySpacedConnector\",\"uuid\":\"f50f8b24-6836-47e2-b898-11b49150a1de\"}],\"packageUris\":[\"http://schema.mathworks.com/mf0/Connector/R2020b\"],\"version\":\"1.0\"}"
  Rotation 312 matrix1 : Subsystem
  A312 : Outport
  angles 312 1 : Outport  Port=2
  wires:
  Rotation 312 matrix1/1(A312) -> A312/1
  Kinematics 312/1(angles) -> Rotation 312 matrix1/1(angles), angles 312 1/1
  angles in/1 -> Kinematics 312/2(angles in)
  w/1 -> Kinematics 312/1(w)
  Enable/1 -> Kinematics 312/3(enabler)

== system Subsystem_repository0x5B10x5D/Euler angles Kinematics /kinematics 323 ==
  w : Inport
  angles_in : Inport  Port=2
  Enable : EnablePort  StatesWhenEnabling=reset  ShowOutputPort=on
  " kinematics 323" : Subsystem
      settings: PortSchema="{\"entries\":[{\"content\":{\"sides\":[{\"content\":{\"connectorIds\":[\"In1\",\"In2\"]},\"type\":\"ConnectorPlacement.EquallySpacedRectSide\",\"uuid\":\"4fd6e809-7da2-4d51-96c7-4627657bb0a7\"},{\"content\":{\"connectorIds\":[\"Out1\"],\"side\":\"RIGHT\"},\"type\":\"ConnectorPlacement.EquallySpacedRectSide\",\"uuid\":\"c66e7720-5f48-4c1c-aaff-2c7b43e45843\"},{\"content\":{\"connectorIds\":[\"In3\"],\"side\":\"TOP\"},\"type\":\"ConnectorPlacement.EquallySpacedRectSide\",\"uuid\":\"5add9d35-dacd-40f3-b2c8-04b7016dc331\"}]},\"type\":\"ConnectorPlacement.EquallySpacedConnector\",\"uuid\":\"f50f8b24-6836-47e2-b898-11b49150a1de\"}],\"packageUris\":[\"http://schema.mathworks.com/mf0/Connector/R2020b\"],\"version\":\"1.0\"}"
  A323 matrix1 : Subsystem
  angles 323 1 : Outport
  A323 : Outport  Port=2
  wires:
  angles_in/1 -> " kinematics 323"/1(angles_in)
  w/1 -> " kinematics 323"/2(w)
  A323 matrix1/1(A323) -> A323/1
  " kinematics 323"/1(angles) -> angles 323 1/1, A323 matrix1/1(angles)
  Enable/1 -> " kinematics 323"/3(enable)

== system Subsystem_repository0x5B10x5D/Euler angles Kinematics /logic 323 ==
  In2 : Inport
  In1 : Inport  Port=2
  AND : Logic  IconShape=distinctive  AllPortsSameDT=off  OutDataTypeStr=boolean
  Clock3 : Clock
  Memory : Memory
  Subsystem4 : Subsystem
  Switch3 : Switch  Criteria=u2 > Threshold  SaturateOnIntegerOverflow=off  InputSameDT=off
  en : Outport
  wires:
  Switch3/1 -> en/1, Memory/1
  Clock3/1 -> Switch3/2
  In1/1 -> Subsystem4/1(In2), AND/1
  In2/1 -> Subsystem4/3(In4), Switch3/3, AND/2
  Subsystem4/1(Out1) -> Switch3/1
  AND/1 -> Subsystem4/2(In1)
  Memory/1 -> Subsystem4/4(In3)

== system Subsystem_repository0x5B10x5D/Euler angles Kinematics /switch 312 ==
  312 angles : Inport
  In1 : Inport  Port=2
  Clock : Clock
  Switch : Switch  Criteria=u2 > Threshold  SaturateOnIntegerOverflow=off  InputSameDT=off
  Out1 : Outport
  wires:
  Switch/1 -> Out1/1
  312 angles/1 -> Switch/1
  Clock/1 -> Switch/2
  In1/1 -> Switch/3

== system Subsystem_repository0x5B10x5D/Euler angles Kinematics /switch enabler 312 ==
  In1 : Inport
  In2 : Inport  Port=2
  Clock1 : Clock
  Switch1 : Switch  Criteria=u2 > Threshold  SaturateOnIntegerOverflow=off  InputSameDT=off
  Out1 : Outport
  wires:
  In2/1 -> Switch1/3
  Clock1/1 -> Switch1/2
  In1/1 -> Switch1/1
  Switch1/1 -> Out1/1

== system Subsystem_repository0x5B10x5D/Gravity gradient Torque/Inertial to LVLH Matrix ==
  n : Inport
  i : Inport  Port=2
  MatrixMultiply : Product  Multiplication=Matrix(*)
  Rotation matrix i : Subsystem
  Rotation matrix n : Subsystem
  A_L/N : Outport
  wires:
  n/1 -> Rotation matrix n/1(n)
  i/1 -> Rotation matrix i/1(i)
  Rotation matrix n/1(R_n) -> MatrixMultiply/1
  Rotation matrix i/1(R_i) -> MatrixMultiply/2
  MatrixMultiply/1 -> A_L/N/1

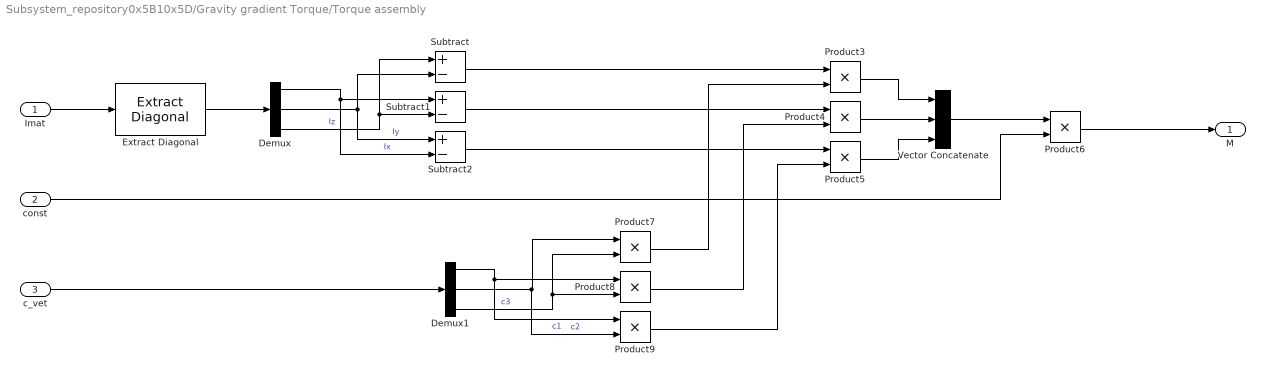
== system Subsystem_repository0x5B10x5D/Gravity gradient Torque/Torque assembly ==
  Imat : Inport
  const : Inport  Port=2
  c_vet : Inport  Port=3
  Demux : Demux  Outputs=3
  Demux1 : Demux  Outputs=3
  Extract Diagonal : matrix_library/Extract Diagonal
      settings: LibrarySourceBlock=|
      | simulink/Matrix
      | Operations/Extract Diagonal
  Product{3..9} (7 alike) : Product
  Subtract : Sum  Inputs=+-
  Subtract1 : Sum  Inputs=+-
  Subtract2 : Sum  Inputs=+-
  Vector Concatenate : Concatenate  NumInputs=3
  M : Outport
  wires:
  Imat/1 -> Extract Diagonal/1
  Extract Diagonal/1 -> Demux/1
  Demux/1 -> Subtract1/1, Subtract2/2  "Ix"
  c_vet/1 -> Demux1/1
  const/1 -> Product6/2
  Demux/2 -> Subtract/2, Subtract2/1  "Iy"
  Demux/3 -> Subtract/1, Subtract1/2  "Iz"
  Product4/1 -> Vector Concatenate/2
  Product3/1 -> Vector Concatenate/1
  Product5/1 -> Vector Concatenate/3
  Vector Concatenate/1 -> Product6/1
  Product6/1 -> M/1
  Demux1/1 -> Product9/1, Product8/1  "c1"
  Demux1/2 -> Product9/2, Product7/1  "c2"
  Demux1/3 -> Product8/2, Product7/2  "c3"
  Product7/1 -> Product3/2
  Product8/1 -> Product4/2
  Product9/1 -> Product5/2
  Subtract/1 -> Product3/1
  Subtract1/1 -> Product4/1
  Subtract2/1 -> Product5/1

== system Subsystem_repository0x5B10x5D/Magnetic field torque/Norm ==
  1 : Inport
  Dot Product : DotProduct  OutDataTypeStr=Inherit: Inherit via internal rule
  Sqrt : Sqrt
  Output : Outport
  wires:
  1/1 -> Dot Product/1, Dot Product/2
  Dot Product/1 -> Sqrt/1
  Sqrt/1 -> Output/1

== system Subsystem_repository0x5B10x5D/Quaternion Kinematics/Matrix creation ==
  In1 : Inport
  Constant : Constant  Value=0
  Demux : Demux  Outputs=3
      settings: DisplayOption=none
  Gain{1..6} (6 alike) : Gain  Gain=-1
  Matrix Concatenate : Concatenate  NumInputs=4  Mode=Multidimensional array  ConcatenateDimension=2
  Vector Concatenate{,1..3} (4 alike) : Concatenate  NumInputs=4
  Out1 : Outport
  wires:
  Gain5/1 -> Vector Concatenate2/1
  Vector Concatenate2/1 -> Matrix Concatenate/3
  Vector Concatenate/1 -> Matrix Concatenate/1
  Gain2/1 -> Vector Concatenate1/3
  Gain4/1 -> Vector Concatenate/2
  Demux/3 -> Vector Concatenate3/3, Gain6/1, Vector Concatenate1/1, Gain4/1  "wz"
  Constant/1 -> Vector Concatenate1/2, Vector Concatenate3/4, Vector Concatenate2/3, Vector Concatenate/1
  Demux/2 -> Vector Concatenate/3, Gain3/1, Vector Concatenate3/2, Gain5/1  "wy"
  Gain1/1 -> Vector Concatenate/4
  Gain3/1 -> Vector Concatenate1/4
  Demux/1 -> Vector Concatenate3/1, Vector Concatenate2/2, Gain2/1, Gain1/1  "wx"
  Gain6/1 -> Vector Concatenate2/4
  Vector Concatenate1/1 -> Matrix Concatenate/2
  Vector Concatenate3/1 -> Matrix Concatenate/4
  In1/1 -> Demux/1
  Matrix Concatenate/1 -> Out1/1

== system Subsystem_repository0x5B10x5D/SRP Torque/Illumination check ==
  1 : Inport
  Constant : Constant  Value=0
  Less Than : RelationalOperator  Operator=<  OutDataTypeStr=boolean  RndMeth=Simplest  InputSameDT=off
  Product6 : Product
  Subtract1 : Sum  Inputs=+-
  Out1 : Outport
  wires:
  1/1 -> Less Than/1, Subtract1/1, Product6/1
  Less Than/1 -> Product6/2
  Product6/1 -> Subtract1/2
  Subtract1/1 -> Out1/1
  Constant/1 -> Less Than/2

== system Subsystem_repository0x5B10x5D/SRP Torque/Normalize ==
  In1 : Inport
  Divide : Product  Inputs=*/
  Divide1 : Product  Inputs=*/
  Divide2 : Product  Inputs=*/
  Selector1 : Selector  NumberOfDimensions=2  InputPortWidth=3  IndexOptions=Index vector (dialog),Index vector (dialog)  Indices=1:N,1  OutputSizes=1,1
  Selector2 : Selector  NumberOfDimensions=2  InputPortWidth=3  IndexOptions=Index vector (dialog),Index vector (dialog)  Indices=1:N,2  OutputSizes=1,1
  Selector6 : Selector  NumberOfDimensions=2  InputPortWidth=3  IndexOptions=Index vector (dialog),Index vector (dialog)  Indices=1:N,3  OutputSizes=1,1
  Sqrt : Sqrt
  Square : Math  Operator=square
  Square1 : Math  Operator=square
  Square2 : Math  Operator=square
  Subtract : Sum  Inputs=+++
  Output : Outport
  Output1 : Outport  Port=2
  Output2 : Outport  Port=3
  wires:
  In1/1 -> Selector1/1, Selector6/1, Selector2/1  "N_b"
  Selector1/1 -> Square/1, Divide/1  "N_b_x"
  Selector2/1 -> Square1/1, Divide1/1  "N_b_y"
  Selector6/1 -> Divide2/1, Square2/1  "N_b_z"
  Square1/1 -> Subtract/2
  Square/1 -> Subtract/1
  Square2/1 -> Subtract/3
  Subtract/1 -> Sqrt/1
  Sqrt/1 -> Divide2/2, Divide/2, Divide1/2
  Divide/1 -> Output/1
  Divide1/1 -> Output1/1
  Divide2/1 -> Output2/1

== system Subsystem_repository0x5B10x5D/Euler angles Kinematics /Subsystem2/check 312_1 ==
  angles 312 : Inport
  Check Static Range : simulink/Model Verification/Check  Static Range  Description=-pi/2+toll <= u <= pi/2 - toll  max=pi/2 - toll  max_included=on  min=-pi/2+toll  min_included=on  enabled=off  stopWhenAssertionFail=off  export=on  icon=graphic
  Selector : Selector  InputPortWidth=3  IndexOptions=Index vector (dialog)  Indices=2  OutputSizes=1
  Out1 : Outport
  wires:
  Check Static Range/1 -> Out1/1
  Selector/1 -> Check Static Range/1
  angles 312/1 -> Selector/1

== system Subsystem_repository0x5B10x5D/Euler angles Kinematics /Subsystem3/If Action Subsystem ==
  In1 : Inport
  Action Port : ActionPort
  Out1 : Outport
  wires:
  In1/1 -> Out1/1

== system Subsystem_repository0x5B10x5D/Euler angles Kinematics /Subsystem3/If Action Subsystem1 ==
  In1 : Inport
  Action Port : ActionPort
  Out1 : Outport
  wires:
  In1/1 -> Out1/1

== system Subsystem_repository0x5B10x5D/Euler angles Kinematics /Subsystem3/If Action Subsystem2 ==
  In1 : Inport
  Action Port : ActionPort
  Out1 : Outport
  wires:
  In1/1 -> Out1/1

== system Subsystem_repository0x5B10x5D/Euler angles Kinematics /Subsystem3/If Action Subsystem3 ==
  In1 : Inport
  Action Port : ActionPort
  Out1 : Outport
  wires:
  In1/1 -> Out1/1

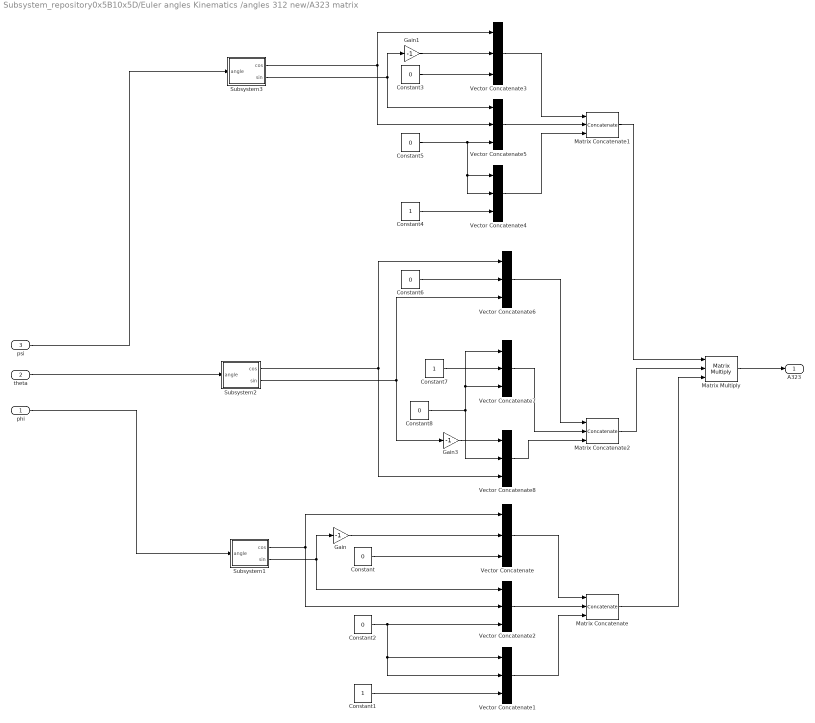
== system Subsystem_repository0x5B10x5D/Euler angles Kinematics /angles 312 new/A323 matrix ==
  phi : Inport
  theta : Inport  Port=2
  psi : Inport  Port=3
  Constant{,2..3,5..6,8} (6 alike) : Constant  Value=0
  Constant1 : Constant
  Constant4 : Constant
  Constant7 : Constant
  Gain : Gain  Gain=-1
  Gain1 : Gain  Gain=-1
  Gain3 : Gain  Gain=-1
  Matrix Concatenate : Concatenate  NumInputs=3  Mode=Multidimensional array  ConcatenateDimension=2
  Matrix Concatenate1 : Concatenate  NumInputs=3  Mode=Multidimensional array  ConcatenateDimension=2
  Matrix Concatenate2 : Concatenate  NumInputs=3  Mode=Multidimensional array  ConcatenateDimension=2
  Matrix Multiply : Product  Inputs=3  Multiplication=Matrix(*)
  Subsystem1 : Subsystem
  Subsystem2 : Subsystem
  Subsystem3 : Subsystem
  Vector Concatenate{,1..8} (9 alike) : Concatenate  NumInputs=3
  A323 : Outport
  wires:
  Subsystem1/2(sin) -> Gain/1, Vector Concatenate2/1
  Subsystem1/1(cos) -> Vector Concatenate2/2, Vector Concatenate/1
  Constant1/1 -> Vector Concatenate1/3
  Gain/1 -> Vector Concatenate/2
  Constant/1 -> Vector Concatenate/3
  Constant2/1 -> Vector Concatenate1/1, Vector Concatenate1/2, Vector Concatenate2/3
  Vector Concatenate/1 -> Matrix Concatenate/1
  Vector Concatenate2/1 -> Matrix Concatenate/2
  Vector Concatenate1/1 -> Matrix Concatenate/3
  Vector Concatenate4/1 -> Matrix Concatenate1/3
  Vector Concatenate5/1 -> Matrix Concatenate1/2
  Vector Concatenate3/1 -> Matrix Concatenate1/1
  Constant5/1 -> Vector Concatenate5/3, Vector Concatenate4/1, Vector Concatenate4/2
  Constant3/1 -> Vector Concatenate3/3
  Gain1/1 -> Vector Concatenate3/2
  Constant4/1 -> Vector Concatenate4/3
  Subsystem3/1(cos) -> Vector Concatenate3/1, Vector Concatenate5/2
  Subsystem3/2(sin) -> Vector Concatenate5/1, Gain1/1
  Matrix Concatenate2/1 -> Matrix Multiply/2
  Matrix Concatenate/1 -> Matrix Multiply/3
  Matrix Concatenate1/1 -> Matrix Multiply/1
  Matrix Multiply/1 -> A323/1
  Vector Concatenate6/1 -> Matrix Concatenate2/1
  Vector Concatenate7/1 -> Matrix Concatenate2/2
  Vector Concatenate8/1 -> Matrix Concatenate2/3
  Subsystem2/1(cos) -> Vector Concatenate8/3, Vector Concatenate6/1
  Constant6/1 -> Vector Concatenate6/2
  Subsystem2/2(sin) -> Vector Concatenate6/3, Gain3/1
  Constant7/1 -> Vector Concatenate7/2
  Constant8/1 -> Vector Concatenate7/1, Vector Concatenate7/3, Vector Concatenate8/2
  Gain3/1 -> Vector Concatenate8/1
  psi/1 -> Subsystem3/1(angle)
  theta/1 -> Subsystem2/1(angle)
  phi/1 -> Subsystem1/1(angle)

== system Subsystem_repository0x5B10x5D/Euler angles Kinematics /angles 312 new/angles_to_312 ==
  A323 : Inport
  Asin : Trigonometry  Operator=asin
  Atan1 : Trigonometry  Operator=atan2
  Atan2 : Trigonometry  Operator=atan2
  Gain : Gain  Gain=-1
  Gain1 : Gain  Gain=-1
  Mux : Mux  Inputs=3
  Selector : Selector  NumberOfDimensions=2  InputPortWidth=3  IndexOptions=Index vector (dialog),Index vector (dialog)  Indices=2,1  OutputSizes=1,1
  Selector1 : Selector  NumberOfDimensions=2  InputPortWidth=3  IndexOptions=Index vector (dialog),Index vector (dialog)  Indices=2,2  OutputSizes=1,1
  Selector2 : Selector  NumberOfDimensions=2  InputPortWidth=3  IndexOptions=Index vector (dialog),Index vector (dialog)  Indices=2,3  OutputSizes=1,1
  Selector3 : Selector  NumberOfDimensions=2  InputPortWidth=3  IndexOptions=Index vector (dialog),Index vector (dialog)  Indices=1,3  OutputSizes=1,1
  Selector4 : Selector  NumberOfDimensions=2  InputPortWidth=3  IndexOptions=Index vector (dialog),Index vector (dialog)  Indices=3,3  OutputSizes=1,1
  312 angles : Outport
  wires:
  Selector/1 -> Gain/1
  Gain/1 -> Atan2/1
  Selector1/1 -> Atan2/2
  Selector2/1 -> Asin/1
  Atan2/1 -> Mux/1
  Asin/1 -> Mux/2
  Mux/1 -> 312 angles/1
  A323/1 -> Selector/1, Selector1/1, Selector3/1, Selector4/1, Selector2/1
  Selector3/1 -> Gain1/1
  Gain1/1 -> Atan1/1
  Selector4/1 -> Atan1/2
  Atan1/1 -> Mux/3

== system Subsystem_repository0x5B10x5D/Euler angles Kinematics /angles 323 new/Rotation 312 matrix2 ==
  phi : Inport
  theta : Inport  Port=2
  psi : Inport  Port=3
  A312 conc : Concatenate  NumInputs=3  Mode=Multidimensional array  ConcatenateDimension=2
  Subsystem : Subsystem
  Subsystem1 : Subsystem
  Subsystem2 : Subsystem
  column 1 : Subsystem
  column 2 : Subsystem
  column 3 : Subsystem
  A312 : Outport
  wires:
  A312 conc/1 -> A312/1
  Subsystem/1(cos) -> column 2/1(phi), column 1/1(phi)
  column 3/1(Out1) -> A312 conc/3
  column 1/1(Out1) -> A312 conc/1
  Subsystem2/2(sin) -> column 3/4(psi2), column 2/6(psi2), column 1/6(psi2)
  column 2/1(Out1) -> A312 conc/2
  Subsystem2/1(cos) -> column 3/3(psi), column 1/5(psi), column 2/5(psi)
  Subsystem1/2(sin) -> column 2/4(theta2), column 1/4(theta2), column 3/2(theta2)
  Subsystem/2(sin) -> column 2/2(phi2), column 1/2(phi2)
  Subsystem1/1(cos) -> column 1/3(theta), column 3/1(theta), column 2/3(theta)
  phi/1 -> Subsystem/1(angle)
  theta/1 -> Subsystem1/1(angle)
  psi/1 -> Subsystem2/1(angle)

== system Subsystem_repository0x5B10x5D/Euler angles Kinematics /angles 323 new/angles_to_323 ==
  A312 : Inport
  Asin : Trigonometry  Operator=acos
  Atan1 : Trigonometry  Operator=atan2
  Atan2 : Trigonometry  Operator=atan2
  Gain2 : Gain  Gain=-1
  Mux : Mux  Inputs=3
  Selector : Selector  NumberOfDimensions=2  InputPortWidth=3  IndexOptions=Index vector (dialog),Index vector (dialog)  Indices=3,2  OutputSizes=1,1
  Selector1 : Selector  NumberOfDimensions=2  InputPortWidth=3  IndexOptions=Index vector (dialog),Index vector (dialog)  Indices=3,1  OutputSizes=1,1
  Selector2 : Selector  NumberOfDimensions=2  InputPortWidth=3  IndexOptions=Index vector (dialog),Index vector (dialog)  Indices=3,3  OutputSizes=1,1
  Selector3 : Selector  NumberOfDimensions=2  InputPortWidth=3  IndexOptions=Index vector (dialog),Index vector (dialog)  Indices=2,3  OutputSizes=1,1
  Selector4 : Selector  NumberOfDimensions=2  InputPortWidth=3  IndexOptions=Index vector (dialog),Index vector (dialog)  Indices=1,3  OutputSizes=1,1
  323 angles : Outport
  wires:
  Mux/1 -> 323 angles/1
  Asin/1 -> Mux/2
  Selector3/1 -> Atan1/1
  Selector4/1 -> Gain2/1
  Atan2/1 -> Mux/1
  Atan1/1 -> Mux/3
  A312/1 -> Selector/1, Selector1/1, Selector3/1, Selector4/1, Selector2/1
  Selector/1 -> Atan2/1
  Selector2/1 -> Asin/1
  Selector1/1 -> Atan2/2
  Gain2/1 -> Atan1/2

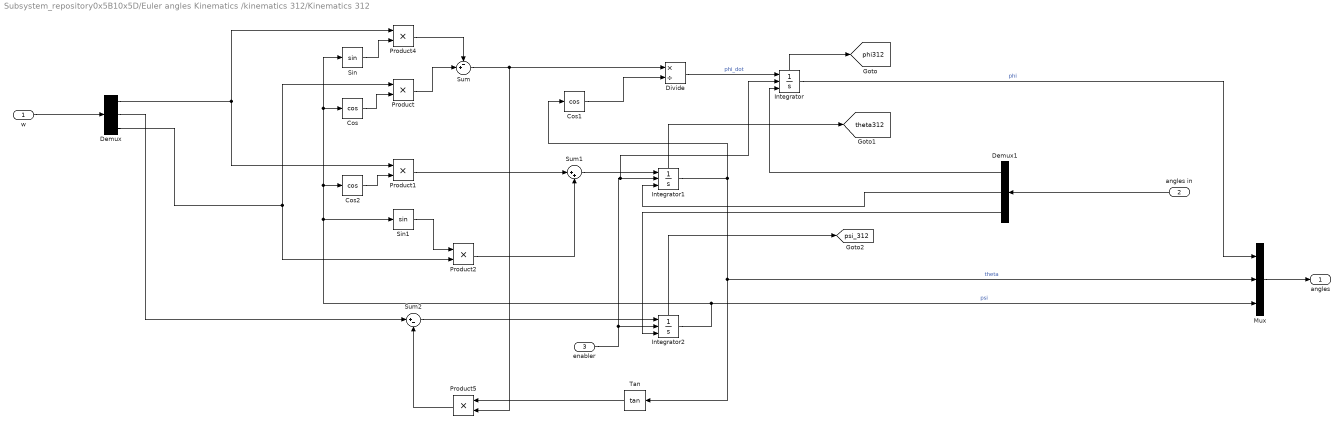
== system Subsystem_repository0x5B10x5D/Euler angles Kinematics /kinematics 312/Kinematics 312 ==
  w : Inport
  angles in : Inport  Port=2
  enabler : Inport  Port=3
  Cos : Trigonometry  Operator=cos
  Cos1 : Trigonometry  Operator=cos
  Cos2 : Trigonometry  Operator=cos
  Demux : Demux  Outputs=3
  Demux1 : Demux  Outputs=3
  Divide : Product  Inputs=*/
  Integrator : Integrator  ExternalReset=rising  InitialConditionSource=external  ShowStatePort=on
  Integrator1 : Integrator  ExternalReset=rising  InitialConditionSource=external  ShowStatePort=on
  Integrator2 : Integrator  ExternalReset=rising  InitialConditionSource=external  ShowStatePort=on  IgnoreLimit=on  ZeroCross=off
  Mux : Mux  Inputs=3
  Product{,1..2,4..5} (5 alike) : Product
  Sin : Trigonometry
  Sin1 : Trigonometry
  Sum : Sum  Inputs=-+|
  Sum1 : Sum  Inputs=|++
  Sum2 : Sum  Inputs=|+-
  Tan : Trigonometry  Operator=tan
  angles : Outport
  tag scope: phi312=global, psi_312=global, theta312=global
  wires:
  Integrator/1 -> Mux/1  "phi"
  Integrator1/1 -> Tan/1, Mux/2, Cos1/1  "theta"
  Integrator2/1 -> Sin/1, Cos/1, Cos2/1, Sin1/1, Mux/3  "psi"
  Cos/1 -> Product/2
  Demux/3 -> Product/1, Product2/2
  Product/1 -> Sum/2
  Sin/1 -> Product4/2
  Demux/1 -> Product4/1, Product1/1
  Cos1/1 -> Divide/2
  Divide/1 -> Integrator/1  "phi_dot"
  Cos2/1 -> Product1/2
  Product1/1 -> Sum1/1
  Sin1/1 -> Product2/1
  Product2/1 -> Sum1/2
  Sum1/1 -> Integrator1/1
  Product4/1 -> Sum/1
  Sum2/1 -> Integrator2/1
  Sum/1 -> Divide/1, Product5/2
  Tan/1 -> Product5/1
  Product5/1 -> Sum2/2
  Demux/2 -> Sum2/1
  w/1 -> Demux/1
  Mux/1 -> angles/1
  angles in/1 -> Demux1/1
  Demux1/1 -> Integrator/3
  Demux1/2 -> Integrator1/3
  Demux1/3 -> Integrator2/3
  enabler/1 -> Integrator/2, Integrator1/2, Integrator2/2
  Integrator/State -> [phi312]
  Integrator1/State -> [theta312]
  Integrator2/State -> [psi_312]

== system Subsystem_repository0x5B10x5D/Euler angles Kinematics /kinematics 312/Rotation 312 matrix1 ==
  angles : Inport
  A312 conc : Concatenate  NumInputs=3  Mode=Multidimensional array  ConcatenateDimension=2
  Demux : Demux  Outputs=3
  Subsystem : Subsystem
  Subsystem1 : Subsystem
  Subsystem2 : Subsystem
  column 1 : Subsystem
  column 2 : Subsystem
  column 3 : Subsystem
  A312 : Outport
  wires:
  angles/1 -> Demux/1
  Subsystem1/1(cos) -> column 2/3(theta), column 3/1(theta), column 1/3(theta)
  Subsystem/2(sin) -> column 1/2(phi2), column 2/2(phi2)
  Subsystem1/2(sin) -> column 3/2(theta2), column 1/4(theta2), column 2/4(theta2)
  Subsystem2/1(cos) -> column 2/5(psi), column 1/5(psi), column 3/3(psi)
  column 2/1(Out1) -> A312 conc/2
  Demux/2 -> Subsystem1/1(angle)
  Subsystem2/2(sin) -> column 1/6(psi2), column 2/6(psi2), column 3/4(psi2)
  Demux/3 -> Subsystem2/1(angle)
  column 1/1(Out1) -> A312 conc/1
  column 3/1(Out1) -> A312 conc/3
  Demux/1 -> Subsystem/1(angle)
  Subsystem/1(cos) -> column 1/1(phi), column 2/1(phi)
  A312 conc/1 -> A312/1

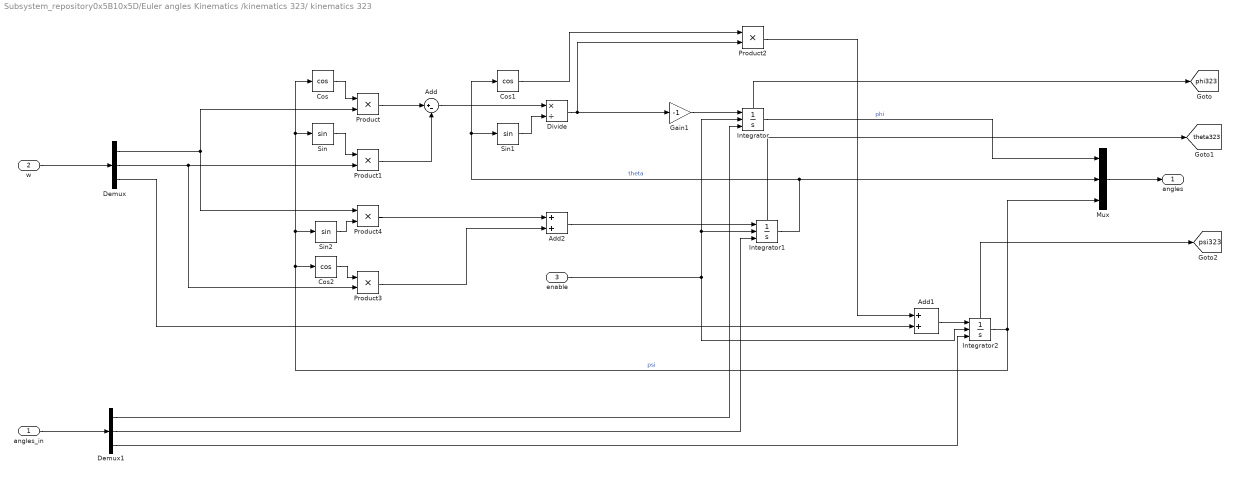
== system Subsystem_repository0x5B10x5D/Euler angles Kinematics /kinematics 323/ kinematics 323 ==
  angles_in : Inport
  w : Inport  Port=2
  enable : Inport  Port=3
  Add : Sum  Inputs=|+-
  Add1 : Sum
  Add2 : Sum
  Cos : Trigonometry  Operator=cos
  Cos1 : Trigonometry  Operator=cos
  Cos2 : Trigonometry  Operator=cos
  Demux : Demux  Outputs=3
  Demux1 : Demux  Outputs=3
  Divide : Product  Inputs=*/
  Gain1 : Gain  Gain=-1
  Integrator : Integrator  ExternalReset=rising  InitialConditionSource=external  ShowStatePort=on
  Integrator1 : Integrator  ExternalReset=rising  InitialConditionSource=external  ShowStatePort=on
  Integrator2 : Integrator  ExternalReset=rising  InitialConditionSource=external  ShowStatePort=on
  Mux : Mux  Inputs=3
  Product{,1..4} (5 alike) : Product
  Sin : Trigonometry
  Sin1 : Trigonometry
  Sin2 : Trigonometry
  angles : Outport
  tag scope: phi323=global, psi323=global, theta323=global
  wires:
  w/1 -> Demux/1
  Integrator2/1 -> Mux/3, Cos/1, Sin/1, Sin2/1, Cos2/1  "psi"
  Integrator1/1 -> Mux/2, Sin1/1, Cos1/1  "theta"
  Integrator/1 -> Mux/1  "phi"
  Demux/1 -> Product4/1, Product/2
  Cos/1 -> Product/1
  Product/1 -> Add/1
  Demux/2 -> Product3/2, Product1/2
  Sin/1 -> Product1/1
  Product1/1 -> Add/2
  Add/1 -> Divide/1
  Sin1/1 -> Divide/2
  Divide/1 -> Gain1/1, Product2/2
  Gain1/1 -> Integrator/1
  Cos1/1 -> Product2/1
  Demux/3 -> Add1/2
  Product2/1 -> Add1/1
  Add1/1 -> Integrator2/1
  Demux1/3 -> Integrator2/3
  Demux1/1 -> Integrator/3
  Cos2/1 -> Product3/1
  Sin2/1 -> Product4/2
  Product4/1 -> Add2/1
  Product3/1 -> Add2/2
  Add2/1 -> Integrator1/1
  Demux1/2 -> Integrator1/3
  Mux/1 -> angles/1
  angles_in/1 -> Demux1/1
  enable/1 -> Integrator/2, Integrator1/2, Integrator2/2
  Integrator/State -> [phi323]
  Integrator1/State -> [theta323]
  Integrator2/State -> [psi323]
